simulink model "u_perf_FlightModel"  (R2018b)
settings: Solver=VariableStepAuto  StartTime=0.0  StopTime=10.0  RelTol=1e-3
libraries: cstblocks x9
settings Model: Creator=nikovertovec  LastModifiedBy=nikovertovec
settings DataIOCC: SaveFinalState=on  SaveState=on

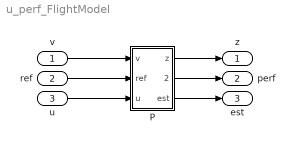
== system u_perf_FlightModel ==
  v : Inport
  ref : Inport  Port=2
  u : Inport  Port=3
  P : Subsystem
  z : Outport
  perf : Outport  Port=2
  est : Outport  Port=3
  wires:
  v/1 -> P/1(v)
  ref/1 -> P/2(ref)
  u/1 -> P/3(u)
  P/1(z) -> z/1
  P/2(perf) -> perf/1
  P/3(est) -> est/1

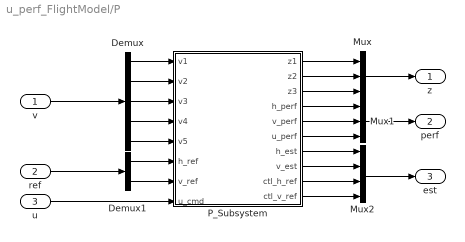
== system u_perf_FlightModel/P ==
  v : Inport
  ref : Inport  Port=2
  u : Inport  Port=3
  Demux : Demux  Outputs=5
  Demux1 : Demux  Outputs=2
  Mux : Mux  Inputs=3
  Mux1 : Mux  Inputs=3
  Mux2 : Mux
  P_Subsystem : Subsystem
  z : Outport
  perf : Outport  Port=2
  est : Outport  Port=3
  wires:
  Mux2/1 -> est/1
  Demux/1 -> P_Subsystem/1(v1)
  ref/1 -> Demux1/1
  Demux1/1 -> P_Subsystem/6(h_ref)
  P_Subsystem/8(v_est) -> Mux2/2
  P_Subsystem/7(h_est) -> Mux2/1
  Demux1/2 -> P_Subsystem/7(v_ref)
  P_Subsystem/5(v_perf) -> Mux1/2
  Demux/5 -> P_Subsystem/5(v5)
  Mux1/1 -> perf/1
  Demux/4 -> P_Subsystem/4(v4)
  Demux/3 -> P_Subsystem/3(v3)
  P_Subsystem/3(z3) -> Mux/3
  P_Subsystem/2(z2) -> Mux/2
  Mux/1 -> z/1
  P_Subsystem/1(z1) -> Mux/1
  P_Subsystem/4(h_perf) -> Mux1/1
  Demux/2 -> P_Subsystem/2(v2)
  u/1 -> P_Subsystem/8(u_cmd)
  v/1 -> Demux/1
  P_Subsystem/9(ctl_h_ref) -> Mux2/3
  P_Subsystem/10(ctl_v_ref) -> Mux2/4
  P_Subsystem/6(u_perf) -> Mux1/3

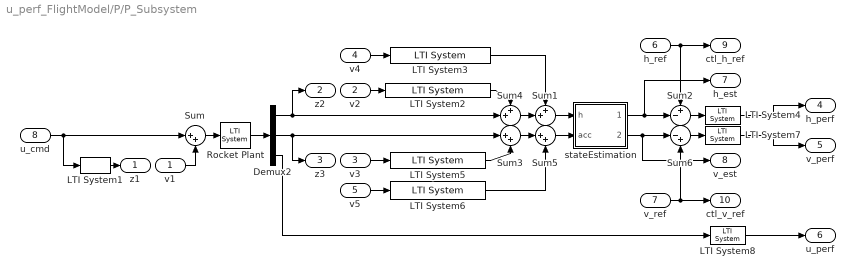
== system u_perf_FlightModel/P/P_Subsystem ==
  v1 : Inport
  v2 : Inport  Port=2
  v3 : Inport  Port=3
  v4 : Inport  Port=4
  v5 : Inport  Port=5
  h_ref : Inport  Port=6
  v_ref : Inport  Port=7
  u_cmd : Inport  Port=8
  Demux2 : Demux  Outputs=3
  LTI System1 : cstblocks/LTI System  sys=Wu  IC=[]
  LTI System2 : cstblocks/LTI System  sys=W_inaccuracies_baro  IC=[]
  LTI System3 : cstblocks/LTI System  sys=W_sensorNoise_baro  IC=[]
  LTI System4 : cstblocks/LTI System  sys=Wp_h  IC=[]
  LTI System5 : cstblocks/LTI System  sys=W_inaccuracies_acc  IC=[]
  LTI System6 : cstblocks/LTI System  sys=W_sensorNoise_acc  IC=[]
  LTI System7 : cstblocks/LTI System  sys=Wp_v  IC=[]
  LTI System8 : cstblocks/LTI System  sys=Wp_u  IC=[]
  Rocket Plant : cstblocks/LTI System  sys=G  IC=[]
  Sum : Sum  Inputs=|++  OutMin=0  OutMax=1
  Sum1 : Sum  Inputs=++|  OutMin=0  OutMax=1
  Sum2 : Sum  Inputs=+-|  OutMin=0  OutMax=1
  Sum3 : Sum  Inputs=|++  OutMin=0  OutMax=1
  Sum4 : Sum  Inputs=++|  OutMin=0  OutMax=1
  Sum5 : Sum  Inputs=|++  OutMin=0  OutMax=1
  Sum6 : Sum  Inputs=|-+  OutMin=0  OutMax=1
  stateEstimation : Subsystem
  z1 : Outport
  z2 : Outport  Port=2
  z3 : Outport  Port=3
  h_perf : Outport  Port=4
  v_perf : Outport  Port=5
  u_perf : Outport  Port=6
  h_est : Outport  Port=7
  v_est : Outport  Port=8
  ctl_h_ref : Outport  Port=9
  ctl_v_ref : Outport  Port=10
  wires:
  v_ref/1 -> Sum6/2, ctl_v_ref/1
  Sum3/1 -> Sum5/1
  Sum1/1 -> stateEstimation/1(h)
  h_ref/1 -> Sum2/1, ctl_h_ref/1
  LTI System3/1 -> Sum1/1
  v2/1 -> LTI System2/1
  Sum4/1 -> Sum1/2
  v5/1 -> LTI System6/1
  LTI System4/1 -> h_perf/1
  v1/1 -> Sum/2
  v4/1 -> LTI System3/1
  LTI System7/1 -> v_perf/1
  Sum6/1 -> LTI System7/1
  stateEstimation/2(v_est) -> v_est/1, Sum6/1
  u_cmd/1 -> LTI System1/1, Sum/1
  LTI System6/1 -> Sum5/2
  LTI System1/1 -> z1/1
  Demux2/2 -> z3/1, Sum3/1
  Sum/1 -> Rocket Plant/1
  LTI System2/1 -> Sum4/1
  LTI System5/1 -> Sum3/2
  stateEstimation/1(h_est) -> h_est/1, Sum2/2
  Demux2/1 -> z2/1, Sum4/2
  Sum2/1 -> LTI System4/1
  v3/1 -> LTI System5/1
  Sum5/1 -> stateEstimation/2(acc)
  Demux2/3 -> LTI System8/1
  Rocket Plant/1 -> Demux2/1
  LTI System8/1 -> u_perf/1

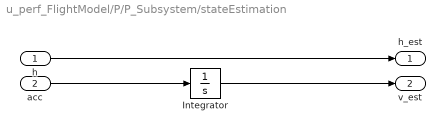
== system u_perf_FlightModel/P/P_Subsystem/stateEstimation ==
  h : Inport
  acc : Inport  Port=2
  Integrator : Integrator
  h_est : Outport
  v_est : Outport  Port=2
  wires:
  acc/1 -> Integrator/1
  h/1 -> h_est/1
  Integrator/1 -> v_est/1
